simulink model "MORUS_NELINEARNI_NELINEARNI_MPC_2"  (R2019a)
settings: Solver=FixedStepAuto  StartTime=0.0  StopTime=sim_time  RelTol=1e-3  EnableMultiTasking=on
values from neighbouring files (symbols this model uses):
  A_dis_calc = expm(kSamplingTime*A_continous_time)    [MPC_designer_X.m]    (also in NonTilting.m; RUN_simulation.m; Simulacija_MPC_YAW_NELINEARNI.m; Simulacija_MPC_Z.m)
  B_dis_calc = integral_exp_A * B_continous_time    [MPC_designer_X.m]    (also in NonTilting.m; RUN_simulation.m; Simulacija_MPC_YAW_NELINEARNI.m; Simulacija_MPC_Z.m)
  b_f = 4.56e-4    (= 0.000456)    [LinearizacijaMatrica.m]    (also in Linearizirane_matrice.mat; MPC_designer_X.m; NonTilting.m; RUN_simulation.m)
  b_m = 0.01    [LinearizacijaMatrica.m]    (also in Linearizirane_matrice.mat; MPC_designer_X.m; NonTilting.m; RUN_simulation.m)
  BETA = 0.0    (= 0)    [LinearizacijaMatrica.m]    (also in Linearizirane_matrice.mat; MPC_designer_X.m; NonTilting.m = 0.200712863979; RUN_simulation.m)
  g = 9.80665    [LinearizacijaMatrica.m]    (also in Linearizirane_matrice.mat; MPC_designer_X.m = 9.81; NonTilting.m = 9.81; RUN_simulation.m = 9.81)
  hover = 427.6233    [MPC_designer_X.m]    (also in NonTilting.m; RUN_simulation.m; Simulacija_MPC_YAW_NELINEARNI.m; Simulacija_MPC_Z.m)
  I_b_xx = 5.5268    [MPC_designer_X.m]    (also in NonTilting.m; RUN_simulation.m; Simulacija_MPC_YAW_NELINEARNI.m; Simulacija_MPC_Z.m)
  I_b_yy = 5.5268    [MPC_designer_X.m]    (also in NonTilting.m; RUN_simulation.m; Simulacija_MPC_YAW_NELINEARNI.m; Simulacija_MPC_Z.m)
  I_b_zz = 6.8854    [MPC_designer_X.m]    (also in NonTilting.m; RUN_simulation.m; Simulacija_MPC_YAW_NELINEARNI.m; Simulacija_MPC_Z.m)
  kSamplingTime = 0.810    (= 0.81)    [MPCDesigner_YAW.m]    (also in MPC_designer_X.m = 0.1; MPC_designer_Z.m; NonTilting.m = 0.015; RUN_simulation.m = 0.015)
  L = 0.84    [LinearizacijaMatrica.m]    (also in Linearizirane_matrice.mat; MPC_designer_X.m; NonTilting.m; RUN_simulation.m)
  m = 1.0    (= 1)    [LinearizacijaMatrica.m]    (also in Linearizirane_matrice.mat; MPC_designer_X.m; NonTilting.m; RUN_simulation.m)
  M = 34.8    [LinearizacijaMatrica.m]    (also in Linearizirane_matrice.mat; MPC_designer_X.m = 34; NonTilting.m = 34; RUN_simulation.m = 34)
  m_b = 30.8    [LinearizacijaMatrica.m]    (also in Linearizirane_matrice.mat; MPC_designer_X.m; NonTilting.m; RUN_simulation.m)
  odabir = 1    [MPC_designer_X.m]    (also in NonTilting.m; RUN_simulation.m; Simulacija_MPC_YAW_NELINEARNI.m; Simulacija_MPC_Z.m)
  polu = 1.0    (= 1)    [Simulacija_Roll.m]
  Q = inv(diag([0.5800 4*kSamplingTime 0.5800 4*kSamplingTime 300 300 0.2 (0.2/3) 100 4])) * diag([0, 0, 0, 0, 0, 0, 1e5,0, 1e7, 0]) *inv(diag([0.5800 4*kSamplingTime 0.5800 4*kSamplingTime 300 300 0.2 (0.2/3.0) 100 4]))    [NonTilting.m]    (also in RUN_simulation.m = diag([ 0.135340000000000,0.002706800000000,  0.1353400, 0.00; Simulacija_MPC_YAW_NELINEARNI.m = diag([pop(5),pop(6),pop(5),pop(6), pop(7),pop(7),pop(8),pop(; Simulacija_MPC_Z.m = diag([pop(5),pop(6),pop(5),pop(6), pop(7),pop(7),pop(8),pop(; Simulacija_Roll.m = diag([pop(5),pop(6),pop(5),pop(6), pop(7),pop(7),pop(8),pop()
  R = inv(diag([0.5800 0.5800 300 300]))*diag([0, 0, 0, 0])*inv(diag([0.5800 0.5800 300 300]))    [NonTilting.m]    (also in RUN_simulation.m = diag([0.67670, 0.67670, 0.13534000, 0.13534000]); Simulacija_MPC_YAW_NELINEARNI.m = diag([pop(1),pop(1),pop(2),pop(2)]); Simulacija_MPC_Z.m = diag([pop(1),pop(1),pop(2),pop(2)]); Simulacija_Roll.m = diag([pop(1),pop(1),pop(2),pop(2)]))
  R_delta = inv(diag([0.5800 0.5800 300 300]))* diag([0,0,0,0])*inv(diag([0.5800 0.5800 300 300]))    [NonTilting.m]    (also in RUN_simulation.m = diag([0.738879858135067, 0.738879858135067, 0.00738879858135; Simulacija_MPC_YAW_NELINEARNI.m = diag([pop(3),pop(3),pop(4),pop(4)]); Simulacija_MPC_Z.m = diag([pop(3),pop(3),pop(4),pop(4)]); Simulacija_Roll.m = diag([pop(3),pop(3),pop(4),pop(4)]))
  T_r = 0.2    [LinearizacijaMatrica.m]    (also in Linearizirane_matrice.mat; MPC_designer_X.m; NonTilting.m; RUN_simulation.m)
  w_mm = 19.7845    [LinearizacijaMatrica.m]    (also in Linearizirane_matrice.mat; MPC_designer_X.m = 17; NonTilting.m = 17; RUN_simulation.m = 17)
  z_m = 0.05    [LinearizacijaMatrica.m]    (also in Linearizirane_matrice.mat; MPC_designer_X.m; NonTilting.m; RUN_simulation.m)
  z_r = 0.2    [LinearizacijaMatrica.m]    (also in Linearizirane_matrice.mat; MPC_designer_X.m; NonTilting.m; RUN_simulation.m)
  zeta_mm = 0.6544    [LinearizacijaMatrica.m]    (also in Linearizirane_matrice.mat; MPC_designer_X.m = 0.85; NonTilting.m = 0.85; RUN_simulation.m = 0.85)
libraries: simulink x6
(part 4 of 5)

== matlab function MORUS_NELINEARNI_NELINEARNI_MPC_2/MPC PITCH/MATLAB Function1 ==
  settings: updateMethod=DISCRETE
  data: x0_ input; u output; x_ss_ input; u_ss_ input; kreni input; A input; B input; R input; R_delta input; Q input; samplingTime input
function u  = adam(x0_, x_ss_, u_ss_, kreni, A, B, R, R_delta, Q, samplingTime)

persistent new_desire_state  pred_horizon control_horizon max_iter     ...
           scale_MV_inv  scale_OV_inv gradients gradient_past ...
           gradient_square_past gradient_past_tilda gradient_square_past_tilda ...
           x_states deriv_wrt_u epsilon rho1 rho2 delta num_heuristic_vars ...
           u_past u_current lambdas_x lambdas_u lambdas_u_ref u_horizon ref_old t u_last_step ...
           du_max u_max x




       
if(isempty(new_desire_state) )
    u_last_step = zeros(4, 1);
    du_max = zeros(4,2);
    u_max = zeros(4,2);
    
    du_max(1,1) = samplingTime * 2;
    du_max(1,2) = -samplingTime * 2;
    du_max(2,1) = samplingTime * 2;
    du_max(2,2) = -samplingTime * 2;
    du_max(3,1) = 1*(samplingTime/0.01);
    du_max(3,2) = -1*(samplingTime/0.01);
    du_max(4,1) = 1*(samplingTime/0.01);
    du_max(4,2) = -1*(samplingTime/0.01);
    
    u_max(1,1) = 0.6 / 2 - 0.01;
    u_max(1,2) = -u_max(1,1);
    u_max(2,1) = 0.6 / 2 - 0.01;
    u_max(2,2) = -u_max(1,1);
    u_max(3,1) = 50;
    u_max(3,2) = -50;
    u_max(4,1) = 50;
    u_max(4,2) = -50;
    
    ref_old  = x_ss_;
    t = 0.0;
    epsilon = 0.03;
	rho1 = 0.9;
	rho2 = 0.999;
	delta = 1e-7;
max_iter = 15;
control_horizon = 5;
pred_horizon = 14;
blocking = [1 2 3 4 4];
pred_hor_block = [];
for cont_iter = 1:control_horizon
    
        for block_iter = 1 : blocking(cont_iter)
            pred_hor_block = [pred_hor_block, cont_iter];
        end
    
end

num_heuristic_vars = 2;
gradients = zeros(num_heuristic_vars*control_horizon,1 );
gradient_past = zeros(num_heuristic_vars*control_horizon,1 );
gradient_past_tilda = zeros(num_heuristic_vars*control_horizon,1 );
gradient_square_past_tilda = zeros(num_heuristic_vars*control_horizon,1 );
gradient_square_past = zeros(num_heuristic_vars*control_horizon,1 );
new_desire_state = true;
scale_OV_inv = inv(diag([0.58, 4.0, 0.58, 4.0, 800, 800, 0.5236, 0.671578600000000]));

scale_MV_inv = inv(diag([0.58, 0.58, 100, 100]));

% R =diag([0.67670, 0.67670, 0.13534000, 0.13534000]);
% R_delta = diag([0.738879858135067, 0.738879858135067, 0.007388798581351,0.007388798581351]);
% Q = diag([ 0.135340000000000,0.002706800000000,  0.1353400, 0.002706800, 0.002706800, 0.002706800,10.7068000, 9.676700]);

% A =[    0.4271,    0.0223,         0,         0,         0,         0,         0 ,        0;
%    -8.7243,   -0.1501,         0,         0,         0,         0,         0,         0;
%          0,         0,    0.4271,    0.0223,         0,         0,         0,         0;
%          0,         0,   -8.7243,   -0.1501,         0,         0,         0,         0;
%          0,         0,         0,         0,    0.7300,         0,         0,         0;
%          0,         0,         0,         0,         0,    0.7300,         0,         0;
%     0.0090,    0.0005,    0.0090,    0.0005,    0.0001,   -0.0001,    1.0000,    0.0787;
%     0.1699,    0.0113,    0.1699,    0.0113,    0.0028,   -0.0028,         0 ,   1.0000];
%     
% B =[ 0.5729,         0 ,        0 ,        0;
%     8.7243,         0   ,      0 ,        0;
%          0,    0.5729  ,       0 ,        0;
%          0,    8.7243 ,        0 ,        0;
%          0,         0 ,   0.2700 ,        0;
%          0,         0 ,        0 ,   0.2700;
%    -0.0037,   -0.0037,    0.0000 ,  -0.0000;
%    -0.0347,   -0.0347,    0.0005 ,  -0.0005];



x_states = zeros(size(A, 1), pred_horizon+1);
deriv_wrt_u =  zeros(size(B,2), control_horizon);
u_past = zeros(size(B,2), 1);
u_current = zeros(size(B,2), 1);
u_ss_ = zeros(size(B,2), 1);
lambdas_x = zeros(size(A, 1), pred_horizon);
lambdas_u = zeros(size(B,2), pred_horizon);
u_horizon = zeros(size(B,2), pred_horizon);
lambdas_u_ref = zeros(size(B,2), pred_horizon);
x = zeros(control_horizon *num_heuristic_vars,1);

end

residuum_signal =0.0;
residuum_state =0.0;

u = zeros(size(B,2), 1);
if(kreni ~= 1)
    return;
end
% x = zeros(control_horizon *num_heuristic_vars,1);

change_x = zeros(control_horizon *num_heuristic_vars,1);

if(sum(abs(x_ss_ - ref_old), 'double') < 1e-6)
   new_desire_state = false; 
else
    new_desire_state = true;
    ref_old = x_ss_;
end
% new_desire_state = false; 
for iter = 1:max_iter
x_states(:,1) = x0_ ;
deriv_wrt_u = 0*deriv_wrt_u;
u_past = zeros(size(B,2), 1);% u_current*1;

if (new_desire_state) 
		new_desire_state = false;
		gradient_past = 0*gradient_past;
		gradient_square_past = 0*gradient_square_past;
        x = zeros(control_horizon *num_heuristic_vars,1);

		t = 0.0;
end

for i = 1:pred_horizon
    if(i <= control_horizon)
        u(1,1) = x(0*control_horizon  + i);
        u(2,1) = x(0*control_horizon  + i);
        u(3,1) = x(1*control_horizon  + i);
        u(4,1) = -x(1*control_horizon  + i);
    end
    x_states(:,i+1) = A * x_states(:,i) + B * u; 
    lambdas_x(:,i) = -1*x_ss_ + x_states(:,i+1); 
    lambdas_u(:,i) = u - u_past; 
    lambdas_u_ref(:, i) = u - u_ss_; 
 
    %derivation of u
    if(i <= control_horizon)
        deriv_wrt_u(:, i) = (2*R*u) -2*R*u_ss_  + (4*R_delta*u) -2*R_delta*u_past + deriv_wrt_u(:, i) ;
        
        if(i > 1)
            deriv_wrt_u(:, i-1) = deriv_wrt_u(:, i-1) -2*R_delta*u ;
        end
    else
        deriv_wrt_u(:, control_horizon) = deriv_wrt_u(:, control_horizon) + (2*R*u) -2*R*u_ss_  + (4*R_delta*u)+ (-2*R_delta*u_past) ;
        deriv_wrt_u(:, control_horizon) = deriv_wrt_u(:, control_horizon) -2*R_delta*u ;
    end
    
    %derivation of x
    for j = 1:i
        if(j <= control_horizon && i <= control_horizon)
            
            deriv_wrt_u(:,j) = deriv_wrt_u(:,j) + transpose(transpose( 2*Q*x_states(:,i+1) - 2*Q*x_ss_ )*(A^(i-j))*B); 
        else
            if(j > control_horizon)
                deriv_wrt_u(:,control_horizon) =deriv_wrt_u(:,control_horizon) +  transpose(transpose((2*Q*x_states(:,i+1) - 2*Q*x_ss_))*(A^(i-j))*B); 
            else
                deriv_wrt_u(:,j) =deriv_wrt_u(:,j) + transpose(transpose( 2*Q*x_states(:,i+1) - 2*Q*x_ss_ )*(A^(i-j))*B); 
            end
        end
    end
    u_past = u;
end


lambdas_u_ref =scale_MV_inv * lambdas_u_ref;
lambdas_u = scale_MV_inv * lambdas_u;
lambdas_x = scale_OV_inv * lambdas_x;
residuum_signal=sum((lambdas_u_ref.*(R*lambdas_u_ref)),'double')  + sum((lambdas_u.*(R_delta*lambdas_u)),'double'); 
residuum_state=sum((lambdas_x.*(Q*lambdas_x)),'double') ; 
        
residuum =  residuum_signal +  residuum_state;

for iter_der = 1:control_horizon
    gradients(iter_der, 1) = 2 * deriv_wrt_u(1, iter_der);
    gradients(iter_der + control_horizon, 1) = 2 * deriv_wrt_u(3, iter_der);
end

gradient_square_past = (rho2*gradient_square_past + (1 - rho2)*gradients.*(gradients));

gradient_past = (rho1*gradient_past + (1 - rho1)*gradients);

t  = t +1.0;

for adam_iter = 1:control_horizon *num_heuristic_vars
    gradient_past_tilda(adam_iter, 1) = (gradient_past(adam_iter, 1)) / (1.0 - (rho1^t));
	gradient_square_past_tilda(adam_iter, 1) = (gradient_square_past(adam_iter, 1)) / (1.0 - (rho2^t));
		

end

for adam_iter = 1:control_horizon *num_heuristic_vars
    change_x(adam_iter, 1) = -1 * (epsilon * gradient_past_tilda(adam_iter, 1)) / (sqrt(gradient_square_past_tilda(adam_iter, 1)) + delta);

end

x = (x + change_x);
end




u(1,1) = x(0*control_horizon  + 1);
u(2,1) = x(0*control_horizon  + 1);
u(3,1) = x(1*control_horizon  + 1);
u(4,1) = -x(1*control_horizon  + 1);

for iter_m = 1:4
    if(u(iter_m,1) > ( u_last_step(iter_m,1)+du_max(iter_m,1) ))
        u(iter_m,1) =  u_last_step(iter_m,1)+du_max(iter_m,1);
        
    elseif (u(iter_m,1) < ( u_last_step(iter_m,1)+du_max(iter_m,2) ))
        u(iter_m,1) =  u_last_step(iter_m,1)+du_max(iter_m,2);
    end
    
    if(u(iter_m,1) > u_max(iter_m,1) )
        u(iter_m,1) =  u_max(iter_m,1);
    elseif (u(iter_m,1) < u_max(iter_m,2))
        u(iter_m,1) =  u_max(iter_m,2);
    end
    
    
end
u_last_step = u;
end

== matlab function MORUS_NELINEARNI_NELINEARNI_MPC_2/MORUS/MATLAB Function ==
  data: ROLL input; DOT_ROLL output; PITCH input; W_X input; W_Y input; W_Z input; DOT_PITCH output; DOT_YAW output
function [DOT_ROLL, DOT_PITCH, DOT_YAW] = fcn(ROLL, PITCH, W_X, W_Y, W_Z)


DOT_ROLL = W_X + sin(ROLL)*tan(PITCH)*W_Y + cos(ROLL)*tan(PITCH)*W_Z;
DOT_PITCH = cos(ROLL)*W_Y -sin(ROLL)*W_Z;
DOT_YAW = (sin(ROLL)/cos(PITCH))*W_Y + (cos(ROLL)/cos(PITCH))*W_Z;

== matlab function MORUS_NELINEARNI_NELINEARNI_MPC_2/MPC ROLL/MATLAB Function2 ==
  settings: updateMethod=DISCRETE
  data: x0_ input; u output; x_ss_ input; u_ss_ input; kreni input; A input; B input; R input; R_delta input; Q input; samplingTime input
function u  = adaGrad(x0_, x_ss_, u_ss_, kreni, A, B,R, R_delta, Q, samplingTime)

persistent new_desire_state  pred_horizon control_horizon max_iter     ...
    scale_MV_inv   scale_OV_inv gradients gradient_past ...
    x_states deriv_wrt_u epsilon delta num_heuristic_vars ...
    u_past u_current lambdas_x lambdas_u lambdas_u_ref u_horizon ref_old t u_last_step ...
    du_max u_max





if(isempty(new_desire_state) )
    u_last_step = zeros(4, 1);
    du_max = zeros(4,2);
    u_max = zeros(4,2);
    
    du_max(1,1) = samplingTime * 2;
    du_max(1,2) = -samplingTime * 2;
    du_max(2,1) = samplingTime * 2;
    du_max(2,2) = -samplingTime * 2;
    du_max(3,1) = 1*(samplingTime/0.01);
    du_max(3,2) = -1*(samplingTime/0.01);
    du_max(4,1) = 1*(samplingTime/0.01);
    du_max(4,2) = -1*(samplingTime/0.01);
    
    u_max(1,1) = 0.6 / 2 - 0.01;
    u_max(1,2) = -u_max(1,1);
    u_max(2,1) = 0.6 / 2 - 0.01;
    u_max(2,2) = -u_max(1,1);
    u_max(3,1) = 50;
    u_max(3,2) = -50;
    u_max(4,1) = 50;
    u_max(4,2) = -50;
    
    ref_old  = x_ss_;
    t = 0.0;
    epsilon = 0.4;
    delta = 1e-7;
    max_iter = 15;
    control_horizon = 5;
    pred_horizon = 14;
    num_heuristic_vars = 2;
    gradients = zeros(num_heuristic_vars*control_horizon,1 );
    gradient_past = zeros(num_heuristic_vars*control_horizon,1 );
    new_desire_state = true;
    scale_OV_inv = inv(diag([0.58, 4.0, 0.58, 4.0, 800, 800, 0.5236, 0.5236]));
    
    scale_MV_inv = inv(diag([0.58, 0.58, 100, 100]));
    
%     R =diag([0.67670, 0.67670, 0.13534000, 0.13534000]);
%     R_delta = diag([0.738879858135067, 0.738879858135067, 0.007388798581351,0.007388798581351]);
%     Q = diag([ 0.135340000000000,0.002706800000000,  0.1353400, 0.002706800, 0.002706800, 0.002706800,10.7068000, 9.676700]);
%     
%     A =[    0.4271,    0.0223,         0,         0,         0,         0,         0 ,        0;
%         -8.7243,   -0.1501,         0,         0,         0,         0,         0,         0;
%         0,         0,    0.4271,    0.0223,         0,         0,         0,         0;
%         0,         0,   -8.7243,   -0.1501,         0,         0,         0,         0;
%         0,         0,         0,         0,    0.7300,         0,         0,         0;
%         0,         0,         0,         0,         0,    0.7300,         0,         0;
%         0.0090,    0.0005,    0.0090,    0.0005,    0.0001,   -0.0001,    1.0000,    0.0787;
%         0.1699,    0.0113,    0.1699,    0.0113,    0.0028,   -0.0028,         0 ,   1.0000];
%     
%     B =[ 0.5729,         0 ,        0 ,        0;
%         8.7243,         0   ,      0 ,        0;
%         0,    0.5729  ,       0 ,        0;
%         0,    8.7243 ,        0 ,        0;
%         0,         0 ,   0.2700 ,        0;
%         0,         0 ,        0 ,   0.2700;
%         -0.0037,   -0.0037,    0.0000 ,  -0.0000;
%         -0.0347,   -0.0347,    0.0005 ,  -0.0005];
    
    
    
    x_states = zeros(size(A, 1), pred_horizon+1);
    deriv_wrt_u =  zeros(size(B,2), control_horizon);
    u_past = zeros(size(B,2), 1);
    u_current = zeros(size(B,2), 1);
    u_ss_ = zeros(size(B,2), 1);
    lambdas_x = zeros(size(A, 1), pred_horizon);
    lambdas_u = zeros(size(B,2), pred_horizon);
    u_horizon = zeros(size(B,2), pred_horizon);
    lambdas_u_ref = zeros(size(B,2), pred_horizon);
    
end

residuum_signal =0.0;
residuum_state =0.0;

u = zeros(size(B,2), 1);

if(kreni ~= 2)
    return
end

x = zeros(control_horizon *num_heuristic_vars,1);
change_x = zeros(control_horizon *num_heuristic_vars,1);

if(sum(abs(x_ss_ - ref_old), 'double') < 1e-6)
    new_desire_state = false;
    
else
    new_desire_state = true;
    ref_old = x_ss_;
end

for iter = 1:max_iter
    x_states(:,1) = x0_ ;
    deriv_wrt_u = 0*deriv_wrt_u;
    u_past = zeros(size(B,2), 1);% u_current*1;
    
    if (new_desire_state)
        new_desire_state = false;
        gradient_past = 0*gradient_past;
    end
    
    for i = 1:pred_horizon
        if(i <= control_horizon)
            u(1,1) = x(0*control_horizon  + i);
            u(2,1) = x(0*control_horizon  + i);
            u(3,1) = x(1*control_horizon  + i);
            u(4,1) = -x(1*control_horizon  + i);
        end
        x_states(:,i+1) = A * x_states(:,i) + B * u;
        lambdas_x(:,i) = -1*x_ss_ + x_states(:,i+1);
        lambdas_u(:,i) = u - u_past;
        lambdas_u_ref(:, i) = u - u_ss_;
        
        %derivation of u
        if(i <= control_horizon)
            deriv_wrt_u(:, i) = (2*R*u) -2*R*u_ss_  + (4*R_delta*u) -2*R_delta*u_past + deriv_wrt_u(:, i) ;
            
            if(i > 1)
                deriv_wrt_u(:, i-1) = deriv_wrt_u(:, i-1) -2*R_delta*u ;
            end
        else
            deriv_wrt_u(:, control_horizon) = deriv_wrt_u(:, control_horizon) + (2*R*u) -2*R*u_ss_  + (4*R_delta*u)+ (-2*R_delta*u_past) ;
            deriv_wrt_u(:, control_horizon) = deriv_wrt_u(:, control_horizon) -2*R_delta*u ;
        end
        
        %derivation of x
        for j = 1:i
            if(j <= control_horizon && i <= control_horizon)
                
                deriv_wrt_u(:,j) = deriv_wrt_u(:,j) + transpose(transpose( 2*Q*x_states(:,i+1) - 2*Q*x_ss_ )*(A^(i-j))*B);
            else
                if(j > control_horizon)
                    deriv_wrt_u(:,control_horizon) =deriv_wrt_u(:,control_horizon) +  transpose(transpose((2*Q*x_states(:,i+1) - 2*Q*x_ss_))*(A^(i-j))*B);
                else
                    deriv_wrt_u(:,j) =deriv_wrt_u(:,j) + transpose(transpose( 2*Q*x_states(:,i+1) - 2*Q*x_ss_ )*(A^(i-j))*B);
                end
            end
        end
        u_past = u;
    end
    
    
    lambdas_u_ref =scale_MV_inv * lambdas_u_ref;
    lambdas_u = scale_MV_inv * lambdas_u;
    lambdas_x = scale_OV_inv * lambdas_x;
    residuum_signal=sum((lambdas_u_ref.*(R*lambdas_u_ref)),'double')  + sum((lambdas_u.*(R_delta*lambdas_u)),'double');
    residuum_state=sum((lambdas_x.*(Q*lambdas_x)),'double') ;
    
    residuum =  residuum_signal +  residuum_state;
    
    for iter_der = 1:control_horizon
        gradients(iter_der, 1) = 2 * deriv_wrt_u(1, iter_der);
        gradients(iter_der + control_horizon, 1) = 2 * deriv_wrt_u(3, iter_der);
    end
    
    
    gradient_past = (gradient_past + gradients.*gradients);
    
    
    
    for adam_iter = 1:control_horizon *num_heuristic_vars
        change_x(adam_iter, 1) = -1 * (epsilon * gradients(adam_iter, 1)) / (sqrt(gradient_past(adam_iter, 1)) + delta);
        
    end
    
    x = (x + change_x);
end

u(1,1) = x(0*control_horizon  + 1);
u(2,1) = x(0*control_horizon  + 1);
u(3,1) = x(1*control_horizon  + 1);
u(4,1) = -x(1*control_horizon  + 1);

for iter_m = 1:4
    if(u(iter_m,1) > ( u_last_step(iter_m,1)+du_max(iter_m,1) ))
        u(iter_m,1) =  u_last_step(iter_m,1)+du_max(iter_m,1);
        
    elseif (u(iter_m,1) < ( u_last_step(iter_m,1)+du_max(iter_m,2) ))
        u(iter_m,1) =  u_last_step(iter_m,1)+du_max(iter_m,2);
    end
    
    if(u(iter_m,1) > u_max(iter_m,1) )
        u(iter_m,1) =  u_max(iter_m,1);
    elseif (u(iter_m,1) < u_max(iter_m,2))
        u(iter_m,1) =  u_max(iter_m,2);
    end
    
    
end
u_last_step = u;
end

== matlab function MORUS_NELINEARNI_NELINEARNI_MPC_2/MPC ROLL/MATLAB Function3 ==
  settings: updateMethod=DISCRETE
  data: x0_ input; u output; x_ss_ input; u_ss_ input; kreni input; A input; B input; R input; R_delta input; Q input; samplingTime input
function u    = RMSProp(x0_, x_ss_, u_ss_, kreni, A, B, R, R_delta, Q, samplingTime)

persistent new_desire_state  pred_horizon control_horizon max_iter     ...
    scale_MV_inv   scale_OV_inv gradients gradient_past ...
    x_states deriv_wrt_u epsilon delta num_heuristic_vars ...
    u_past u_current lambdas_x lambdas_u lambdas_u_ref u_horizon ref_old t u_last_step ...
    du_max u_max  rho residuum_old 

residuum = 0;


if(isempty(new_desire_state) )
    residuum_old = 1e5;
    u_last_step = zeros(4, 1);
    du_max = zeros(4,2);
    u_max = zeros(4,2);
    
    du_max(1,1) = samplingTime * 2;
    du_max(1,2) = -samplingTime * 2;
    du_max(2,1) = samplingTime * 2;
    du_max(2,2) = -samplingTime * 2;
    du_max(3,1) = 1*(samplingTime/0.01);
    du_max(3,2) = -1*(samplingTime/0.01);
    du_max(4,1) = 1*(samplingTime/0.01);
    du_max(4,2) = -1*(samplingTime/0.01);
    rho = 0.999;
    u_max(1,1) = 0.6 / 2 - 0.01;
    u_max(1,2) = -u_max(1,1);
    u_max(2,1) = 0.6 / 2 - 0.01;
    u_max(2,2) = -u_max(1,1);
    u_max(3,1) = 50;
    u_max(3,2) = -50;
    u_max(4,1) = 50;
    u_max(4,2) = -50;
    
    ref_old  = x_ss_;
    t = 0.0;
    epsilon = 0.4;
    delta = 1e-7;
    max_iter = 15;
    control_horizon = 5;
    pred_horizon = 14;
    num_heuristic_vars = 2;
    gradients = zeros(num_heuristic_vars*control_horizon,1 );
    gradient_past = zeros(num_heuristic_vars*control_horizon,1 );
    new_desire_state = true;
    scale_OV_inv = inv(diag([0.58, 4.0, 0.58, 4.0, 800, 800, 0.5236, 0.5236]));
    
    scale_MV_inv = inv(diag([0.58, 0.58, 100, 100]));
%     
%     R =diag([0.67670, 0.67670, 0.13534000, 0.13534000]);
%     R_delta = diag([0.738879858135067, 0.738879858135067, 0.007388798581351,0.007388798581351]);
%     Q = diag([ 0.135340000000000,0.002706800000000,  0.1353400, 0.002706800, 0.002706800, 0.002706800,10.7068000, 9.676700]);
%     
%     A =[    0.4271,    0.0223,         0,         0,         0,         0,         0 ,        0;
%         -8.7243,   -0.1501,         0,         0,         0,         0,         0,         0;
%         0,         0,    0.4271,    0.0223,         0,         0,         0,         0;
%         0,         0,   -8.7243,   -0.1501,         0,         0,         0,         0;
%         0,         0,         0,         0,    0.7300,         0,         0,         0;
%         0,         0,         0,         0,         0,    0.7300,         0,         0;
%         0.0090,    0.0005,    0.0090,    0.0005,    0.0001,   -0.0001,    1.0000,    0.0787;
%         0.1699,    0.0113,    0.1699,    0.0113,    0.0028,   -0.0028,         0 ,   1.0000];
%     
%     B =[ 0.5729,         0 ,        0 ,        0;
%         8.7243,         0   ,      0 ,        0;
%         0,    0.5729  ,       0 ,        0;
%         0,    8.7243 ,        0 ,        0;
%         0,         0 ,   0.2700 ,        0;
%         0,         0 ,        0 ,   0.2700;
%         -0.0037,   -0.0037,    0.0000 ,  -0.0000;
%         -0.0347,   -0.0347,    0.0005 ,  -0.0005];
    
    
    
    x_states = zeros(size(A, 1), pred_horizon+1);
    deriv_wrt_u =  zeros(size(B,2), control_horizon);
    u_past = zeros(size(B,2), 1);
    u_current = zeros(size(B,2), 1);
    u_ss_ = zeros(size(B,2), 1);
    lambdas_x = zeros(size(A, 1), pred_horizon);
    lambdas_u = zeros(size(B,2), pred_horizon);
    u_horizon = zeros(size(B,2), pred_horizon);
    lambdas_u_ref = zeros(size(B,2), pred_horizon);
    
end

residuum_signal =0.0;
residuum_state =0.0;

u = zeros(size(B,2), 1);
if(kreni ~= 3)
    return
end
x = zeros(control_horizon *num_heuristic_vars,1);
change_x = zeros(control_horizon *num_heuristic_vars,1);

if(sum(sum(abs(x_ss_ - ref_old), 'double')) < 1e-6)
    new_desire_state = false;
    
else
    new_desire_state = true;
    ref_old = x_ss_;
end
if (new_desire_state)
        new_desire_state = false;
        gradient_past = 0*gradient_past;
        residuum_old = 1e5;
end

if(residuum_old < 1e-4)
    return;
end

for iter = 1:max_iter
    x_states(:,1) = x0_ ;
    deriv_wrt_u = 0*deriv_wrt_u;
    u_past = zeros(size(B,2), 1);% u_current*1;
    
    
    
    for i = 1:pred_horizon
        if(i <= control_horizon)
            u(1,1) = x(0*control_horizon  + i);
            u(2,1) = x(0*control_horizon  + i);
            u(3,1) = x(1*control_horizon  + i);
            u(4,1) = -x(1*control_horizon  + i);
        end
        x_states(:,i+1) = A * x_states(:,i) + B * u;
        lambdas_x(:,i) = -1*x_ss_ + x_states(:,i+1);
        lambdas_u(:,i) = u - u_past;
        lambdas_u_ref(:, i) = u - u_ss_;
        
        %derivation of u
        if(i <= control_horizon)
            deriv_wrt_u(:, i) = (2*R*u) -2*R*u_ss_  + (4*R_delta*u) -2*R_delta*u_past + deriv_wrt_u(:, i) ;
            
            if(i > 1)
                deriv_wrt_u(:, i-1) = deriv_wrt_u(:, i-1) -2*R_delta*u ;
            end
        else
            deriv_wrt_u(:, control_horizon) = deriv_wrt_u(:, control_horizon) + (2*R*u) -2*R*u_ss_  + (4*R_delta*u)+ (-2*R_delta*u_past) ;
            deriv_wrt_u(:, control_horizon) = deriv_wrt_u(:, control_horizon) -2*R_delta*u ;
        end
        
        %derivation of x
        for j = 1:i
            if(j <= control_horizon && i <= control_horizon)
                
                deriv_wrt_u(:,j) = deriv_wrt_u(:,j) + transpose(transpose( 2*Q*x_states(:,i+1) - 2*Q*x_ss_ )*(A^(i-j))*B);
            else
                if(j > control_horizon)
                    deriv_wrt_u(:,control_horizon) =deriv_wrt_u(:,control_horizon) +  transpose(transpose((2*Q*x_states(:,i+1) - 2*Q*x_ss_))*(A^(i-j))*B);
                else
                    deriv_wrt_u(:,j) =deriv_wrt_u(:,j) + transpose(transpose( 2*Q*x_states(:,i+1) - 2*Q*x_ss_ )*(A^(i-j))*B);
                end
            end
        end
        u_past = u;
    end
    
    
    lambdas_u_ref =scale_MV_inv * lambdas_u_ref;
    lambdas_u = scale_MV_inv * lambdas_u;
    lambdas_x = scale_OV_inv * lambdas_x;
    residuum_signal=sum(sum((lambdas_u_ref.*(R*lambdas_u_ref)),'double'))  + sum(sum((lambdas_u.*(R_delta*lambdas_u)),'double'));
    residuum_state=sum(sum((lambdas_x.*(Q*lambdas_x)),'double')) ;
    
    residuum =  residuum_signal +  residuum_state;
    
    
    
    for iter_der = 1:control_horizon
        gradients(iter_der, 1) = 2 * deriv_wrt_u(1, iter_der);
        gradients(iter_der + control_horizon, 1) = 2 * deriv_wrt_u(3, iter_der);
    end
    
    
    gradient_past = (rho*gradient_past + (1-rho)*gradients.*gradients);
    
    
    
    for adam_iter = 1:control_horizon *num_heuristic_vars
        change_x(adam_iter, 1) = -1 * (epsilon * gradients(adam_iter, 1)) / (sqrt(gradient_past(adam_iter, 1)) + delta);
        
    end
    
    x = (x + change_x);
end

u(1,1) = x(0*control_horizon  + 1);
u(2,1) = x(0*control_horizon  + 1);
u(3,1) = x(1*control_horizon  + 1);
u(4,1) = -x(1*control_horizon  + 1);

for iter_m = 1:4
    if(u(iter_m,1) > ( u_last_step(iter_m,1)+du_max(iter_m,1) ))
        u(iter_m,1) =  u_last_step(iter_m,1)+du_max(iter_m,1);
        
    elseif (u(iter_m,1) < ( u_last_step(iter_m,1)+du_max(iter_m,2) ))
        u(iter_m,1) =  u_last_step(iter_m,1)+du_max(iter_m,2);
    end
    
    if(u(iter_m,1) > u_max(iter_m,1) )
        u(iter_m,1) =  u_max(iter_m,1);
    elseif (u(iter_m,1) < u_max(iter_m,2))
        u(iter_m,1) =  u_max(iter_m,2);
    end
    
    
end
if(residuum_old < residuum)
    u = 0*u;
    return;
end
u_last_step = u;
residuum_old = residuum;
end

== matlab function MORUS_NELINEARNI_NELINEARNI_MPC_2/MPC ROLL/MATLAB Function4 ==
  settings: updateMethod=DISCRETE
  data: x0_ input; u output; x_ss_ input; u_ss_ input; kreni input; A input; B input; R input; R_delta input; Q input; samplingTime input
function u   = RMSPropNester(x0_, x_ss_, u_ss_, kreni, A, B, R, R_delta, Q, samplingTime)

persistent new_desire_state  pred_horizon control_horizon max_iter    ...
    scale_MV_inv   scale_OV_inv gradients gradient_past ...
    x_states deriv_wrt_u epsilon delta num_heuristic_vars ...
    u_past u_current lambdas_x lambdas_u lambdas_u_ref u_horizon ref_old t u_last_step ...
    du_max u_max  rho residuum_old alpha change_x x

residuum = 0;


if(isempty(new_desire_state) )
    residuum_old = 1e25;
    u_last_step = zeros(4, 1);
    du_max = zeros(4,2);
    u_max = zeros(4,2);
    alpha = 200;
    du_max(1,1) = samplingTime * 2;
    du_max(1,2) = -samplingTime * 2;
    du_max(2,1) = samplingTime * 2;
    du_max(2,2) = -samplingTime * 2;
    du_max(3,1) = 1*(samplingTime/0.01);
    du_max(3,2) = -1*(samplingTime/0.01);
    du_max(4,1) = 1*(samplingTime/0.01);
    du_max(4,2) = -1*(samplingTime/0.01);
    rho = 0.999;
    u_max(1,1) = 0.6 / 2 - 0.01;
    u_max(1,2) = -u_max(1,1);
    u_max(2,1) = 0.6 / 2 - 0.01;
    u_max(2,2) = -u_max(1,1);
    u_max(3,1) = 50;
    u_max(3,2) = -50;
    u_max(4,1) = 50;
    u_max(4,2) = -50;
    
    ref_old  = x_ss_;
    t = 0.0;
    epsilon = 0.4;
    delta = 1e-7;
    max_iter = 15;
    control_horizon = 5;
    pred_horizon = 14;
    num_heuristic_vars = 2;
    gradients = zeros(num_heuristic_vars*control_horizon,1 );
    gradient_past = zeros(num_heuristic_vars*control_horizon,1 );
    new_desire_state = true;
    scale_OV_inv = inv(diag([0.58, 4.0, 0.58, 4.0, 800, 800, 0.5236, 0.5236]));
    
    scale_MV_inv = inv(diag([0.58, 0.58, 100, 100]));
    
%     R =diag([0.67670, 0.67670, 0.13534000, 0.13534000]);
%     R_delta = diag([0.738879858135067, 0.738879858135067, 0.007388798581351,0.007388798581351]);
%     Q = diag([ 0.135340000000000,0.002706800000000,  0.1353400, 0.002706800, 0.002706800, 0.002706800,10.7068000, 9.676700]);
%     
%     A =[    0.4271,    0.0223,         0,         0,         0,         0,         0 ,        0;
%         -8.7243,   -0.1501,         0,         0,         0,         0,         0,         0;
%         0,         0,    0.4271,    0.0223,         0,         0,         0,         0;
%         0,         0,   -8.7243,   -0.1501,         0,         0,         0,         0;
%         0,         0,         0,         0,    0.7300,         0,         0,         0;
%         0,         0,         0,         0,         0,    0.7300,         0,         0;
%         0.0090,    0.0005,    0.0090,    0.0005,    0.0001,   -0.0001,    1.0000,    0.0787;
%         0.1699,    0.0113,    0.1699,    0.0113,    0.0028,   -0.0028,         0 ,   1.0000];
%     
%     B =[ 0.5729,         0 ,        0 ,        0;
%         8.7243,         0   ,      0 ,        0;
%         0,    0.5729  ,       0 ,        0;
%         0,    8.7243 ,        0 ,        0;
%         0,         0 ,   0.2700 ,        0;
%         0,         0 ,        0 ,   0.2700;
%         -0.0037,   -0.0037,    0.0000 ,  -0.0000;
%         -0.0347,   -0.0347,    0.0005 ,  -0.0005];
    
    
    
    x_states = zeros(size(A, 1), pred_horizon+1);
    deriv_wrt_u =  zeros(size(B,2), control_horizon);
    u_past = zeros(size(B,2), 1);
    u_current = zeros(size(B,2), 1);
    u_ss_ = zeros(size(B,2), 1);
    lambdas_x = zeros(size(A, 1), pred_horizon);
    lambdas_u = zeros(size(B,2), pred_horizon);
    u_horizon = zeros(size(B,2), pred_horizon);
    lambdas_u_ref = zeros(size(B,2), pred_horizon);
    change_x = zeros(control_horizon *num_heuristic_vars,1);
    x = zeros(control_horizon *num_heuristic_vars,1);

    
end

residuum_signal =0.0;
residuum_state =0.0;

u = zeros(size(B,2), 1);
if(kreni ~= 4)
    return
end
change_x = zeros(control_horizon *num_heuristic_vars,1);

if(sum(sum(abs(x_ss_ - ref_old), 'double')) < 1e-6)
    new_desire_state = false;
    
else
    new_desire_state = true;
    ref_old = x_ss_;
end
if (new_desire_state)
        new_desire_state = false;
        gradient_past = 0*gradient_past;
        residuum_old = 1e25;
        alpha = 200;
        x = zeros(control_horizon *num_heuristic_vars,1);

end

if(residuum_old < 1e-4)
    return;
end

for iter = 1:max_iter
    x_states(:,1) = x0_ ;
    deriv_wrt_u = 0*deriv_wrt_u;
    u_past = zeros(size(B,2), 1);% u_current*1;
    
    
    x_tilda = x + alpha * change_x;
    for i = 1:pred_horizon
        if(i <= control_horizon)
            u(1,1) = x_tilda(0*control_horizon  + i);
            u(2,1) = x_tilda(0*control_horizon  + i);
            u(3,1) = x_tilda(1*control_horizon  + i);
            u(4,1) = -x_tilda(1*control_horizon  + i);
        end
        x_states(:,i+1) = A * x_states(:,i) + B * u;
        lambdas_x(:,i) = -1*x_ss_ + x_states(:,i+1);
        lambdas_u(:,i) = u - u_past;
        lambdas_u_ref(:, i) = u - u_ss_;
        
        %derivation of u
        if(i <= control_horizon)
            deriv_wrt_u(:, i) = (2*R*u) -2*R*u_ss_  + (4*R_delta*u) -2*R_delta*u_past + deriv_wrt_u(:, i) ;
            
            if(i > 1)
                deriv_wrt_u(:, i-1) = deriv_wrt_u(:, i-1) -2*R_delta*u ;
            end
        else
            deriv_wrt_u(:, control_horizon) = deriv_wrt_u(:, control_horizon) + (2*R*u) -2*R*u_ss_  + (4*R_delta*u)+ (-2*R_delta*u_past) ;
            deriv_wrt_u(:, control_horizon) = deriv_wrt_u(:, control_horizon) -2*R_delta*u ;
        end
        
        %derivation of x
        for j = 1:i
            if(j <= control_horizon && i <= control_horizon)
                
                deriv_wrt_u(:,j) = deriv_wrt_u(:,j) + transpose(transpose( 2*Q*x_states(:,i+1) - 2*Q*x_ss_ )*(A^(i-j))*B);
            else
                if(j > control_horizon)
                    deriv_wrt_u(:,control_horizon) =deriv_wrt_u(:,control_horizon) +  transpose(transpose((2*Q*x_states(:,i+1) - 2*Q*x_ss_))*(A^(i-j))*B);
                else
                    deriv_wrt_u(:,j) =deriv_wrt_u(:,j) + transpose(transpose( 2*Q*x_states(:,i+1) - 2*Q*x_ss_ )*(A^(i-j))*B);
                end
            end
        end
        u_past = u;
    end
    
    
    lambdas_u_ref =scale_MV_inv * lambdas_u_ref;
    lambdas_u = scale_MV_inv * lambdas_u;
    lambdas_x = scale_OV_inv * lambdas_x;
    residuum_signal=sum(sum((lambdas_u_ref.*(R*lambdas_u_ref)),'double'))  + sum(sum((lambdas_u.*(R_delta*lambdas_u)),'double'));
    residuum_state=sum(sum((lambdas_x.*(Q*lambdas_x)),'double')) ;
    
    residuum =  residuum_signal +  residuum_state;
    if(residuum < 0.1)
        alpha = 1e-5;
    end
    
    
    for iter_der = 1:control_horizon
        gradients(iter_der, 1) = 2 * deriv_wrt_u(1, iter_der);
        gradients(iter_der + control_horizon, 1) = 2 * deriv_wrt_u(3, iter_der);
    end
    
    
    gradient_past = (rho*gradient_past + (1-rho)*gradients.*gradients);
    
    
    
    for adam_iter = 1:control_horizon *num_heuristic_vars
        change_x(adam_iter, 1) =alpha * change_x(adam_iter, 1)  -1 * (epsilon * gradients(adam_iter, 1)) / (sqrt(gradient_past(adam_iter, 1)) + delta);
        
    end
    
    x = (x + change_x);
end

u(1,1) = x(0*control_horizon  + 1);
u(2,1) = x(0*control_horizon  + 1);
u(3,1) = x(1*control_horizon  + 1);
u(4,1) = -x(1*control_horizon  + 1);

for iter_m = 1:4
    if(u(iter_m,1) > ( u_last_step(iter_m,1)+du_max(iter_m,1) ))
        u(iter_m,1) =  u_last_step(iter_m,1)+du_max(iter_m,1);
        
    elseif (u(iter_m,1) < ( u_last_step(iter_m,1)+du_max(iter_m,2) ))
        u(iter_m,1) =  u_last_step(iter_m,1)+du_max(iter_m,2);
    end
    
    if(u(iter_m,1) > u_max(iter_m,1) )
        u(iter_m,1) =  u_max(iter_m,1);
    elseif (u(iter_m,1) < u_max(iter_m,2))
        u(iter_m,1) =  u_max(iter_m,2);
    end
    
    
end
if(residuum_old < residuum)
    u = 0*u;
    return;
end
u_last_step = u;
residuum_old = residuum;
end

== matlab function MORUS_NELINEARNI_NELINEARNI_MPC_2/MPC PITCH/MATLAB Function2 ==
  settings: updateMethod=DISCRETE
  data: x0_ input; u output; x_ss_ input; u_ss_ input; kreni input; A input; B input; R input; R_delta input; Q input; samplingTime input
function u  = adaGrad(x0_, x_ss_, u_ss_, kreni, A, B,R, R_delta, Q, samplingTime)

persistent new_desire_state  pred_horizon control_horizon max_iter     ...
    scale_MV_inv   scale_OV_inv gradients gradient_past ...
    x_states deriv_wrt_u epsilon delta num_heuristic_vars ...
    u_past u_current lambdas_x lambdas_u lambdas_u_ref u_horizon ref_old t u_last_step ...
    du_max u_max





if(isempty(new_desire_state) )
    u_last_step = zeros(4, 1);
    du_max = zeros(4,2);
    u_max = zeros(4,2);
    
    du_max(1,1) = samplingTime * 2;
    du_max(1,2) = -samplingTime * 2;
    du_max(2,1) = samplingTime * 2;
    du_max(2,2) = -samplingTime * 2;
    du_max(3,1) = 1*(samplingTime/0.01);
    du_max(3,2) = -1*(samplingTime/0.01);
    du_max(4,1) = 1*(samplingTime/0.01);
    du_max(4,2) = -1*(samplingTime/0.01);
    
    u_max(1,1) = 0.6 / 2 - 0.01;
    u_max(1,2) = -u_max(1,1);
    u_max(2,1) = 0.6 / 2 - 0.01;
    u_max(2,2) = -u_max(1,1);
    u_max(3,1) = 50;
    u_max(3,2) = -50;
    u_max(4,1) = 50;
    u_max(4,2) = -50;
    
    ref_old  = x_ss_;
    t = 0.0;
    epsilon = 0.4;
    delta = 1e-7;
    max_iter = 15;
    control_horizon = 5;
    pred_horizon = 14;
    num_heuristic_vars = 2;
    gradients = zeros(num_heuristic_vars*control_horizon,1 );
    gradient_past = zeros(num_heuristic_vars*control_horizon,1 );
    new_desire_state = true;
    scale_OV_inv = inv(diag([0.58, 4.0, 0.58, 4.0, 800, 800, 0.5236, 0.5236]));
    
    scale_MV_inv = inv(diag([0.58, 0.58, 100, 100]));
    
%     R =diag([0.67670, 0.67670, 0.13534000, 0.13534000]);
%     R_delta = diag([0.738879858135067, 0.738879858135067, 0.007388798581351,0.007388798581351]);
%     Q = diag([ 0.135340000000000,0.002706800000000,  0.1353400, 0.002706800, 0.002706800, 0.002706800,10.7068000, 9.676700]);
%     
%     A =[    0.4271,    0.0223,         0,         0,         0,         0,         0 ,        0;
%         -8.7243,   -0.1501,         0,         0,         0,         0,         0,         0;
%         0,         0,    0.4271,    0.0223,         0,         0,         0,         0;
%         0,         0,   -8.7243,   -0.1501,         0,         0,         0,         0;
%         0,         0,         0,         0,    0.7300,         0,         0,         0;
%         0,         0,         0,         0,         0,    0.7300,         0,         0;
%         0.0090,    0.0005,    0.0090,    0.0005,    0.0001,   -0.0001,    1.0000,    0.0787;
%         0.1699,    0.0113,    0.1699,    0.0113,    0.0028,   -0.0028,         0 ,   1.0000];
%     
%     B =[ 0.5729,         0 ,        0 ,        0;
%         8.7243,         0   ,      0 ,        0;
%         0,    0.5729  ,       0 ,        0;
%         0,    8.7243 ,        0 ,        0;
%         0,         0 ,   0.2700 ,        0;
%         0,         0 ,        0 ,   0.2700;
%         -0.0037,   -0.0037,    0.0000 ,  -0.0000;
%         -0.0347,   -0.0347,    0.0005 ,  -0.0005];
    
    
    
    x_states = zeros(size(A, 1), pred_horizon+1);
    deriv_wrt_u =  zeros(size(B,2), control_horizon);
    u_past = zeros(size(B,2), 1);
    u_current = zeros(size(B,2), 1);
    u_ss_ = zeros(size(B,2), 1);
    lambdas_x = zeros(size(A, 1), pred_horizon);
    lambdas_u = zeros(size(B,2), pred_horizon);
    u_horizon = zeros(size(B,2), pred_horizon);
    lambdas_u_ref = zeros(size(B,2), pred_horizon);
    
end

residuum_signal =0.0;
residuum_state =0.0;

u = zeros(size(B,2), 1);

if(kreni ~= 2)
    return
end

x = zeros(control_horizon *num_heuristic_vars,1);
change_x = zeros(control_horizon *num_heuristic_vars,1);

if(sum(abs(x_ss_ - ref_old), 'double') < 1e-6)
    new_desire_state = false;
    
else
    new_desire_state = true;
    ref_old = x_ss_;
end

for iter = 1:max_iter
    x_states(:,1) = x0_ ;
    deriv_wrt_u = 0*deriv_wrt_u;
    u_past = zeros(size(B,2), 1);% u_current*1;
    
    if (new_desire_state)
        new_desire_state = false;
        gradient_past = 0*gradient_past;
    end
    
    for i = 1:pred_horizon
        if(i <= control_horizon)
            u(1,1) = x(0*control_horizon  + i);
            u(2,1) = x(0*control_horizon  + i);
            u(3,1) = x(1*control_horizon  + i);
            u(4,1) = -x(1*control_horizon  + i);
        end
        x_states(:,i+1) = A * x_states(:,i) + B * u;
        lambdas_x(:,i) = -1*x_ss_ + x_states(:,i+1);
        lambdas_u(:,i) = u - u_past;
        lambdas_u_ref(:, i) = u - u_ss_;
        
        %derivation of u
        if(i <= control_horizon)
            deriv_wrt_u(:, i) = (2*R*u) -2*R*u_ss_  + (4*R_delta*u) -2*R_delta*u_past + deriv_wrt_u(:, i) ;
            
            if(i > 1)
                deriv_wrt_u(:, i-1) = deriv_wrt_u(:, i-1) -2*R_delta*u ;
            end
        else
            deriv_wrt_u(:, control_horizon) = deriv_wrt_u(:, control_horizon) + (2*R*u) -2*R*u_ss_  + (4*R_delta*u)+ (-2*R_delta*u_past) ;
            deriv_wrt_u(:, control_horizon) = deriv_wrt_u(:, control_horizon) -2*R_delta*u ;
        end
        
        %derivation of x
        for j = 1:i
            if(j <= control_horizon && i <= control_horizon)
                
                deriv_wrt_u(:,j) = deriv_wrt_u(:,j) + transpose(transpose( 2*Q*x_states(:,i+1) - 2*Q*x_ss_ )*(A^(i-j))*B);
            else
                if(j > control_horizon)
                    deriv_wrt_u(:,control_horizon) =deriv_wrt_u(:,control_horizon) +  transpose(transpose((2*Q*x_states(:,i+1) - 2*Q*x_ss_))*(A^(i-j))*B);
                else
                    deriv_wrt_u(:,j) =deriv_wrt_u(:,j) + transpose(transpose( 2*Q*x_states(:,i+1) - 2*Q*x_ss_ )*(A^(i-j))*B);
                end
            end
        end
        u_past = u;
    end
    
    
    lambdas_u_ref =scale_MV_inv * lambdas_u_ref;
    lambdas_u = scale_MV_inv * lambdas_u;
    lambdas_x = scale_OV_inv * lambdas_x;
    residuum_signal=sum((lambdas_u_ref.*(R*lambdas_u_ref)),'double')  + sum((lambdas_u.*(R_delta*lambdas_u)),'double');
    residuum_state=sum((lambdas_x.*(Q*lambdas_x)),'double') ;
    
    residuum =  residuum_signal +  residuum_state;
    
    for iter_der = 1:control_horizon
        gradients(iter_der, 1) = 2 * deriv_wrt_u(1, iter_der);
        gradients(iter_der + control_horizon, 1) = 2 * deriv_wrt_u(3, iter_der);
    end
    
    
    gradient_past = (gradient_past + gradients.*gradients);
    
    
    
    for adam_iter = 1:control_horizon *num_heuristic_vars
        change_x(adam_iter, 1) = -1 * (epsilon * gradients(adam_iter, 1)) / (sqrt(gradient_past(adam_iter, 1)) + delta);
        
    end
    
    x = (x + change_x);
end

u(1,1) = x(0*control_horizon  + 1);
u(2,1) = x(0*control_horizon  + 1);
u(3,1) = x(1*control_horizon  + 1);
u(4,1) = -x(1*control_horizon  + 1);

for iter_m = 1:4
    if(u(iter_m,1) > ( u_last_step(iter_m,1)+du_max(iter_m,1) ))
        u(iter_m,1) =  u_last_step(iter_m,1)+du_max(iter_m,1);
        
    elseif (u(iter_m,1) < ( u_last_step(iter_m,1)+du_max(iter_m,2) ))
        u(iter_m,1) =  u_last_step(iter_m,1)+du_max(iter_m,2);
    end
    
    if(u(iter_m,1) > u_max(iter_m,1) )
        u(iter_m,1) =  u_max(iter_m,1);
    elseif (u(iter_m,1) < u_max(iter_m,2))
        u(iter_m,1) =  u_max(iter_m,2);
    end
    
    
end
u_last_step = u;
end
